simulink model "PID_braking_system_A28"  (Simulink 8.5)
settings: Solver=ode45  StartTime=0.0  StopTime=20.0  RelTol=1e-3
libraries: simulink x1
settings Model: Creator=MrPiccolo  LastModifiedBy=MrPiccolo
settings DataIOCC: SignalLoggingSaveFormat=Dataset
settings OptimizationCC: ExpressionDepthLimit=128
settings DebuggingCC: UnderspecifiedInitializationDetection=Simplified  MergeDetectMultiDrivingBlocksExec=error  FcnCallInpInsideContextMsg=EnableAllAsError  StateNameClashWarn=none
settings GRTTargetCC: CombineOutputUpdateFcns=on  GRTInterface=off

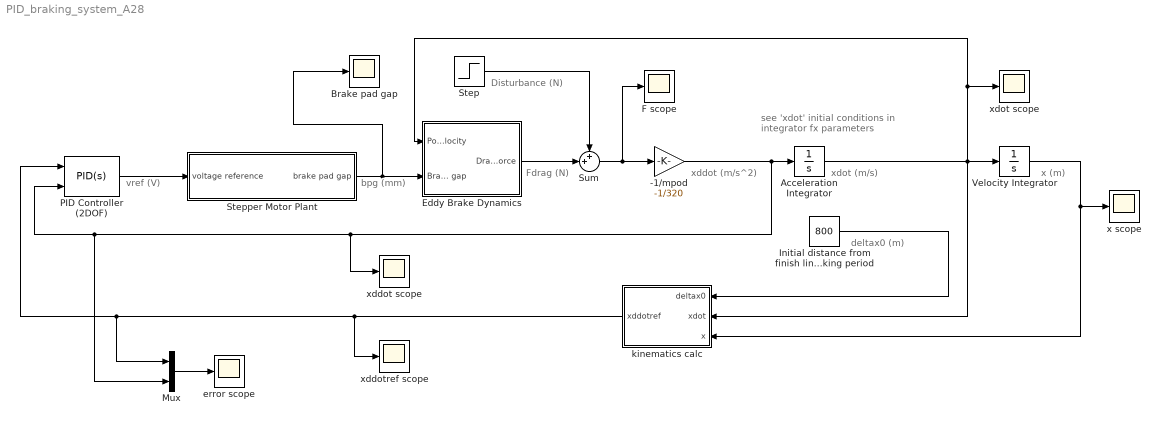
== system PID_braking_system_A28 ==
  note: Fdrag (N)
  note: xddot (m/s^2)
  note: xdot (m/s)
  note: Disturbance (N)
  note: x (m)
  note: deltax0 (m)
  note: vref (V)
  note: bpg (mm)
  note: see 'xdot' initial conditions
      | in integrator fx parameters
  -1/mpod : Gain  Gain=-1/320
  Acceleration Integrator : Integrator  InitialCondition=120
  Brake pad gap : Scope
      settings: SaveName=ScopeData6
  Eddy Brake Dynamics : Subsystem
  F scope : Scope
      settings: SaveName=ScopeData5
  Initial distance from finish line at start of braking period : Constant  Value=800
  Mux : Mux  Inputs=2
  PID Controller (2DOF) : simulink/Continuous/PID Controller (2DOF)  Controller=PID  TimeDomain=Continuous-time  SampleTime=-1  IntegratorMethod=Forward Euler  FilterMethod=Forward Euler  Form=Parallel  UseFilter=on  ControllerParametersSource=internal  P=1  I=1  D=0  N=100  b=1  c=1  InitialConditionSource=internal  InitialConditionForIntegrator=0  InitialConditionForFilter=0  ExternalReset=none  LimitOutput=off  UpperSaturationLimit=inf  LowerSaturationLimit=-inf  LinearizeAsGain=on  AntiWindupMode=none  Kb=1  TrackingMode=off  Kt=1  PParamMin=[]  PParamMax=[]  IParamMin=[]  IParamMax=[]  DParamMin=[]  DParamMax=[]  NParamMin=[]  NParamMax=[]  bParamMin=[]  bParamMax=[]  cParamMin=[]  cParamMax=[]  KbParamMin=[]  KbParamMax=[]  KtParamMin=[]  KtParamMax=[]  POutMin=[]  POutMax=[]  IOutMin=[]  IOutMax=[]  DOutMin=[]  DOutMax=[]  NOutMin=[]  NOutMax=[]  bOutMin=[]  bOutMax=[]  cOutMin=[]  cOutMax=[]  KbOutMin=[]  KbOutMax=[]  KtOutMin=[]  KtOutMax=[]  IntegratorOutMin=[]  IntegratorOutMax=[]  FilterOutMin=[]  FilterOutMax=[]  SumOutMin=[]  SumOutMax=[]  Sum1OutMin=[]  Sum1OutMax=[]  Sum2OutMin=[]  Sum2OutMax=[]  Sum3OutMin=[]  Sum3OutMax=[]  SumI1OutMin=[]  SumI1OutMax=[]  SumI2OutMin=[]  SumI2OutMax=[]  SumI3OutMin=[]  SumI3OutMax=[]  SumDOutMin=[]  SumDOutMax=[]  SaturationOutMin=[]  SaturationOutMax=[]  IntegratorContinuousStateAttributes=''  IntegratorStateMustResolveToSignalObject=off  IntegratorRTWStateStorageClass=Auto  FilterContinuousStateAttributes=''  FilterStateMustResolveToSignalObject=off  FilterRTWStateStorageClass=Auto  DifferentiatorICPrevScaledInput=0  DifferentiatorOutMin=[]  DifferentiatorOutMax=[]
  Step : Step  SampleTime=0
  Stepper Motor Plant : Subsystem
  Sum : Sum  Inputs=++|
  Velocity Integrator : Integrator
  error scope : Scope
      settings: SaveName=ScopeData2
  kinematics calc : Subsystem
  x scope : Scope
      settings: YMin=0  YMax=6000
  xddot scope : Scope
      settings: SaveName=ScopeData4
  xddotref scope : Scope
      settings: SaveName=ScopeData3
  xdot scope : Scope
  wires:
  Eddy Brake Dynamics/1(Drag Force) -> Sum/2
  Step/1 -> Sum/1
  Sum/1 -> F scope/1, -1/mpod/1
  -1/mpod/1 -> xddot scope/1, Mux/2, PID Controller (2DOF)/2, Acceleration Integrator/1
  Acceleration Integrator/1 -> Velocity Integrator/1, xdot scope/1, Eddy Brake Dynamics/1(Pod velocity), kinematics calc/2(xdot)
  Initial distance from finish line at start of braking period/1 -> kinematics calc/1(deltax0)
  Velocity Integrator/1 -> x scope/1, kinematics calc/3(x)
  kinematics calc/1(xddotref) -> xddotref scope/1, Mux/1, PID Controller (2DOF)/1
  PID Controller (2DOF)/1 -> Stepper Motor Plant/1(voltage reference)
  Stepper Motor Plant/1(brake pad gap) -> Brake pad gap/1, Eddy Brake Dynamics/2(Brake pad gap)
  Mux/1 -> error scope/1

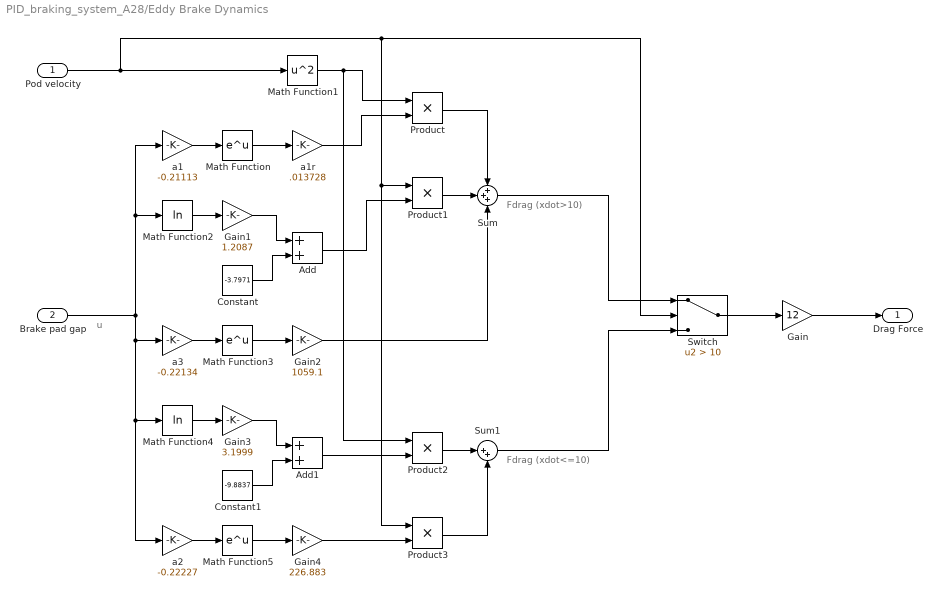
== system PID_braking_system_A28/Eddy Brake Dynamics ==
  note: Fdrag (xdot>10)
  note: u
  note: Fdrag (xdot<=10)
  Pod velocity : Inport
  Brake pad gap : Inport  Port=2
  Add : Sum
  Add1 : Sum
  Constant : Constant  Value=-3.7971
  Constant1 : Constant  Value=-9.8837
  Gain : Gain  Gain=12
  Gain1 : Gain  Gain=1.2087
  Gain2 : Gain  Gain=1059.1
  Gain3 : Gain  Gain=3.1999
  Gain4 : Gain  Gain=226.883
  Math Function : Math  SaturateOnIntegerOverflow=on
  Math Function1 : Math  Operator=square  SaturateOnIntegerOverflow=on
  Math Function2 : Math  Operator=log  SaturateOnIntegerOverflow=on
  Math Function3 : Math  SaturateOnIntegerOverflow=on
  Math Function4 : Math  Operator=log  SaturateOnIntegerOverflow=on
  Math Function5 : Math  SaturateOnIntegerOverflow=on
  Product{,1..3} (4 alike) : Product
  Sum : Sum  Inputs=+++
  Sum1 : Sum  Inputs=|++
  Switch : Switch  Criteria=u2 > Threshold  Threshold=10
  a1 : Gain  Gain=-0.21113
  a1r : Gain  Gain=.013728
  a2 : Gain  Gain=-0.22227
  a3 : Gain  Gain=-0.22134
  Drag Force : Outport
  wires:
  a1/1 -> Math Function/1
  Product/1 -> Sum/1
  Math Function/1 -> a1r/1
  Math Function1/1 -> Product2/1, Product/1
  Math Function2/1 -> Gain1/1
  Product1/1 -> Sum/2
  Brake pad gap/1 -> Math Function2/1, a1/1, a2/1, Math Function4/1, a3/1
  a3/1 -> Math Function3/1
  a1r/1 -> Product/2
  Math Function3/1 -> Gain2/1
  Gain2/1 -> Sum/3
  Pod velocity/1 -> Switch/2, Product3/1, Product1/1, Math Function1/1
  Gain1/1 -> Add/1
  Add/1 -> Product1/2
  Constant/1 -> Add/2
  Sum/1 -> Switch/1
  Math Function4/1 -> Gain3/1
  Gain3/1 -> Add1/1
  Constant1/1 -> Add1/2
  a2/1 -> Math Function5/1
  Math Function5/1 -> Gain4/1
  Sum1/1 -> Switch/3
  Product3/1 -> Sum1/2
  Product2/1 -> Sum1/1
  Add1/1 -> Product2/2
  Gain4/1 -> Product3/2
  Switch/1 -> Gain/1
  Gain/1 -> Drag Force/1

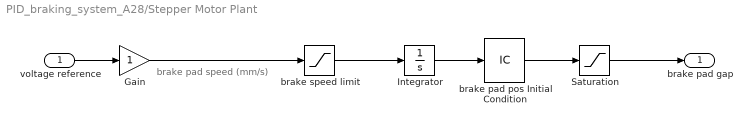
== system PID_braking_system_A28/Stepper Motor Plant ==
  note: brake pad speed (mm/s)
  voltage reference : Inport
  Gain : Gain
  Integrator : Integrator
  Saturation : Saturate  UpperLimit=25  LowerLimit=2.5
  brake pad pos Initial Condition : InitialCondition  Value=25
  brake speed limit : Saturate  UpperLimit=15  LowerLimit=0
  brake pad gap : Outport
  wires:
  voltage reference/1 -> Gain/1
  Gain/1 -> brake speed limit/1
  Integrator/1 -> brake pad pos Initial Condition/1
  Saturation/1 -> brake pad gap/1
  brake pad pos Initial Condition/1 -> Saturation/1
  brake speed limit/1 -> Integrator/1

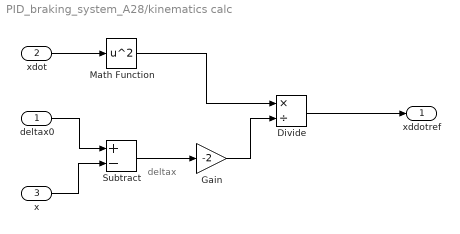
== system PID_braking_system_A28/kinematics calc ==
  note: deltax
  deltax0 : Inport
  xdot : Inport  Port=2
  x : Inport  Port=3
  Divide : Product  Inputs=*/
  Gain : Gain  Gain=-2
  Math Function : Math  Operator=square  SaturateOnIntegerOverflow=on
  Subtract : Sum  Inputs=+-
  xddotref : Outport
  wires:
  x/1 -> Subtract/2
  deltax0/1 -> Subtract/1
  Subtract/1 -> Gain/1
  xdot/1 -> Math Function/1
  Gain/1 -> Divide/2
  Math Function/1 -> Divide/1
  Divide/1 -> xddotref/1
